simulink model "SimulinkModelExample"  (R2015a)
settings: Solver=ode3  StartTime=0.0  StopTime=4  FixedStep=0.001  RelTol=1e-3
libraries: simulink x3
settings Model: Creator=balsi  LastModifiedBy=balsi

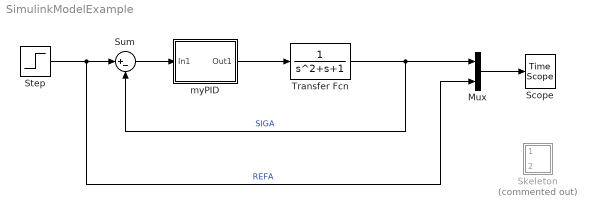
== system SimulinkModelExample ==
  Mux : Mux  Inputs=2
  Scope : TimeScope
  Skeleton : Subsystem  Commented=on
  Step : Step  After=10  SampleTime=0
  Sum : Sum  Inputs=|+-
  Transfer Fcn : TransferFcn  Denominator=[1 1 1]
  myPID : Subsystem
  wires:
  Step/1 -> Mux/2, Sum/1  "REFA"
  Mux/1 -> Scope/1
  myPID/1(Out1) -> Transfer Fcn/1
  Transfer Fcn/1 -> Mux/1, Sum/2  "SIGA"
  Sum/1 -> myPID/1(In1)

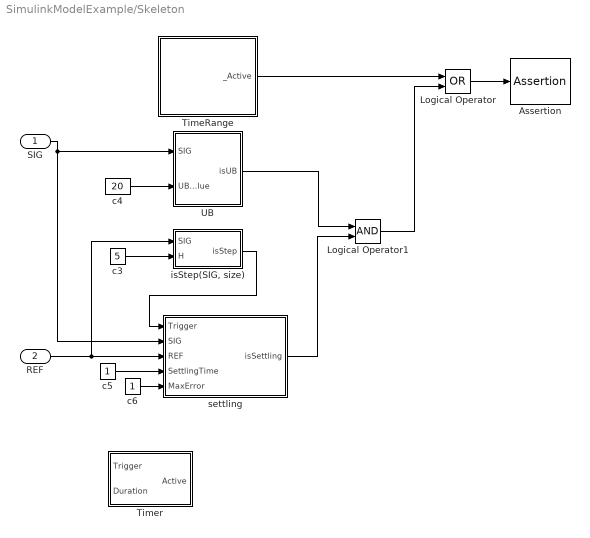
== system SimulinkModelExample/Skeleton ==
  SIG : Inport
  REF : Inport  Port=2
  Assertion : Assertion
  Logical Operator : Logic  Operator=OR  AllPortsSameDT=off  OutDataTypeStr=boolean
  Logical Operator1 : Logic  AllPortsSameDT=off  OutDataTypeStr=boolean
  TimeRange : Subsystem
  Timer : Subsystem
  UB : Subsystem
  c3 : Constant  Value=5
  c4 : Constant  Value=20
  c5 : Constant
  c6 : Constant
  "isStep(SIG, size)" : Subsystem
  settling : Subsystem
  wires:
  SIG/1 -> settling/2(SIG), UB/1(SIG)
  c3/1 -> "isStep(SIG, size)"/2(H)
  "isStep(SIG, size)"/1(isStep) -> settling/1(Trigger)
  c4/1 -> UB/2(UBvalue)
  UB/1(isUB) -> Logical Operator1/1
  REF/1 -> "isStep(SIG, size)"/1(SIG), settling/3(REF)
  c5/1 -> settling/4(SettlingTime)
  c6/1 -> settling/5(MaxError)
  settling/1(isSettling) -> Logical Operator1/2
  Logical Operator1/1 -> Logical Operator/2
  TimeRange/1(_Active) -> Logical Operator/1
  Logical Operator/1 -> Assertion/1

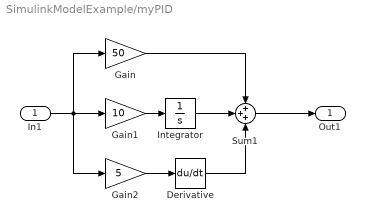
== system SimulinkModelExample/myPID ==
  In1 : Inport
  Derivative : Derivative
  Gain : Gain  Gain=50
  Gain1 : Gain  Gain=10
  Gain2 : Gain  Gain=5
  Integrator : Integrator
  Sum1 : Sum  Inputs=+++
  Out1 : Outport
  wires:
  Derivative/1 -> Sum1/3
  Integrator/1 -> Sum1/2
  Gain/1 -> Sum1/1
  In1/1 -> Gain2/1, Gain/1, Gain1/1
  Sum1/1 -> Out1/1
  Gain1/1 -> Integrator/1
  Gain2/1 -> Derivative/1

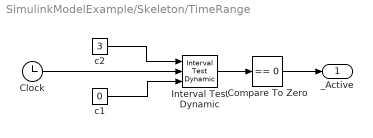
== system SimulinkModelExample/Skeleton/TimeRange ==
  Clock : Clock
  Compare To Zero : simulink/Logic and Bit Operations/Compare To Zero  relop===  OutDataTypeStr=boolean
  Interval Test Dynamic : simulink/Logic and Bit Operations/Interval Test Dynamic  IntervalClosedRight=on  IntervalClosedLeft=on  OutDataTypeStr=boolean
  c1 : Constant  Value=0
  c2 : Constant  Value=3
  _Active : Outport
  wires:
  c1/1 -> Interval Test Dynamic/3
  Clock/1 -> Interval Test Dynamic/2
  c2/1 -> Interval Test Dynamic/1
  Interval Test Dynamic/1 -> Compare To Zero/1
  Compare To Zero/1 -> _Active/1

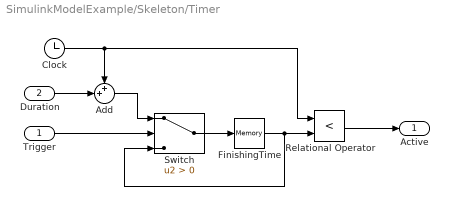
== system SimulinkModelExample/Skeleton/Timer ==
  Trigger : Inport
  Duration : Inport  Port=2
  Add : Sum  Inputs=++|
  Clock : Clock
  FinishingTime : Memory
  Relational Operator : RelationalOperator  Operator=<  OutDataTypeStr=boolean
  Switch : Switch  Criteria=u2 > Threshold
  Active : Outport
  wires:
  Clock/1 -> Relational Operator/1, Add/1
  FinishingTime/1 -> Switch/3, Relational Operator/2
  Relational Operator/1 -> Active/1
  Switch/1 -> FinishingTime/1
  Trigger/1 -> Switch/2
  Duration/1 -> Add/2
  Add/1 -> Switch/1

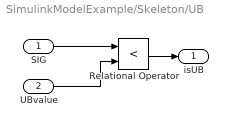
== system SimulinkModelExample/Skeleton/UB ==
  SIG : Inport
  UBvalue : Inport  Port=2
  Relational Operator : RelationalOperator  Operator=<  OutDataTypeStr=boolean
  isUB : Outport
  wires:
  SIG/1 -> Relational Operator/1
  Relational Operator/1 -> isUB/1
  UBvalue/1 -> Relational Operator/2

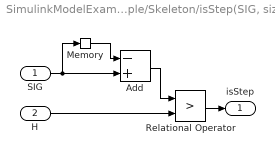
== system SimulinkModelExample/Skeleton/isStep(SIG, size) ==
  SIG : Inport
  H : Inport  Port=2
  Add : Sum  Inputs=-+
  Memory : Memory
  Relational Operator : RelationalOperator  Operator=>  OutDataTypeStr=boolean
  isStep : Outport
  wires:
  Relational Operator/1 -> isStep/1
  SIG/1 -> Add/2, Memory/1
  H/1 -> Relational Operator/2
  Memory/1 -> Add/1
  Add/1 -> Relational Operator/1

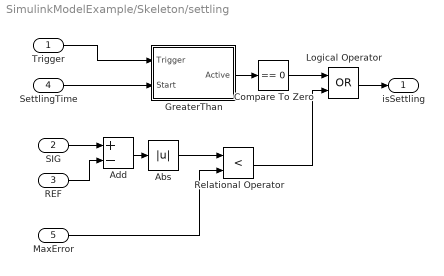
== system SimulinkModelExample/Skeleton/settling ==
  Trigger : Inport
  SIG : Inport  Port=2
  REF : Inport  Port=3
  SettlingTime : Inport  Port=4
  MaxError : Inport  Port=5
  Abs : Abs
  Add : Sum  Inputs=+-
  Compare To Zero : simulink/Logic and Bit Operations/Compare To Zero  relop===  OutDataTypeStr=boolean
  GreaterThan : Subsystem
  Logical Operator : Logic  Operator=OR  AllPortsSameDT=off  OutDataTypeStr=boolean
  Relational Operator : RelationalOperator  Operator=<  OutDataTypeStr=boolean
  isSettling : Outport
  wires:
  Trigger/1 -> GreaterThan/1(Trigger)
  SIG/1 -> Add/1
  REF/1 -> Add/2
  Add/1 -> Abs/1
  Abs/1 -> Relational Operator/1
  Relational Operator/1 -> Logical Operator/2
  MaxError/1 -> Relational Operator/2
  Logical Operator/1 -> isSettling/1
  SettlingTime/1 -> GreaterThan/2(Start)
  GreaterThan/1(Active) -> Compare To Zero/1
  Compare To Zero/1 -> Logical Operator/1

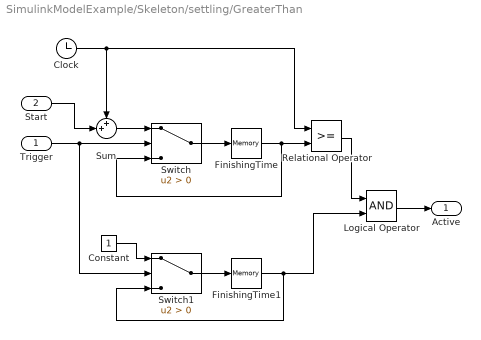
== system SimulinkModelExample/Skeleton/settling/GreaterThan ==
  Trigger : Inport
  Start : Inport  Port=2
  Clock : Clock
  Constant : Constant
  FinishingTime : Memory
  FinishingTime1 : Memory
  Logical Operator : Logic  AllPortsSameDT=off  OutDataTypeStr=boolean
  Relational Operator : RelationalOperator  OutDataTypeStr=boolean
  Sum : Sum  Inputs=++|
  Switch : Switch  Criteria=u2 > Threshold
  Switch1 : Switch  Criteria=u2 > Threshold
  Active : Outport
  wires:
  Clock/1 -> Sum/1, Relational Operator/1
  FinishingTime/1 -> Relational Operator/2, Switch/3
  Relational Operator/1 -> Logical Operator/1
  Switch/1 -> FinishingTime/1
  Trigger/1 -> Switch1/2, Switch/2
  Start/1 -> Sum/2
  Sum/1 -> Switch/1
  Logical Operator/1 -> Active/1
  Switch1/1 -> FinishingTime1/1
  FinishingTime1/1 -> Switch1/3, Logical Operator/2
  Constant/1 -> Switch1/1
